simulink model "pendule_inverse"  (R2020b)
settings: Solver=ode5  StartTime=0.0  StopTime=20  FixedStep=0.1  RelTol=1e-3  EnableMultiTasking=on
values from neighbouring files (symbols this model uses):
  A = [ 0 1     0     0 ... (first row only)    [script_Labo4.m]
  B = [ 0 1/M 0 1/(M*l) ]'    [script_Labo4.m]
  g = 9.81    [script_Labo4.m]
  l = 0.5    [script_Labo4.m]
  m = 1    [script_Labo4.m]
  M = 1    [script_Labo4.m]
undefined symbols (not defined in the file or in its folder): Kd1, Kd2, Kp1, Kp2
settings Model: Creator=Administrateur  LastModifiedBy=dsaussie
settings SolverCC: AutoInsertRateTranBlk=on
settings DataIOCC: LimitDataPoints=on  SaveFormat=Array  SignalLoggingSaveFormat=ModelDataLogs  ReturnWorkspaceOutputs=off
settings OptimizationCC: ExpressionDepthLimit=2147483647  InitFltsAndDblsToZero=on  LifeSpan=inf
settings DebuggingCC: UnderspecifiedInitializationDetection=Classic  MergeDetectMultiDrivingBlocksExec=none  SolverPrmCheckMsg=warning  FcnCallInpInsideContextMsg=warning  StateNameClashWarn=warning  SFUnexpectedBacktrackingDiag=warning  SFNoUnconditionalDefaultTransitionDiag=warning  SFExecutionAtInitializationDiag=none  ArithmeticOperatorsInVariantConditions=warning
settings HardwareCC: ProdBitPerPointer=32  ProdBitPerSizeT=32  ProdBitPerPtrDiffT=32  ProdLargestAtomicFloat=None  ProdIntDivRoundTo=Undefined  ProdEndianess=Unspecified  ProdWordSize=32  ProdHWDeviceType=32-bit Generic
settings ModelReferenceCC: PropagateSignalLabelsOutOfModel=off
settings SFSimCC: SimUseLocalCustomCode=off  CustomCodeUndefinedFunction=UseInterfaceOnly
settings RTWCC: RTWUseLocalCustomCode=off
settings CodeAppCC: StateflowObjectComments=on
settings GRTTargetCC: TargetLangStandard=C89/C90 (ANSI)  CombineOutputUpdateFcns=off  GRTInterface=on
settings ConfigComp: CovMetricSettings=dw  CovSaveCumulativeToWorkspaceVar=on  CovSaveSingleToWorkspaceVar=on  CovExternalEMLEnable=off

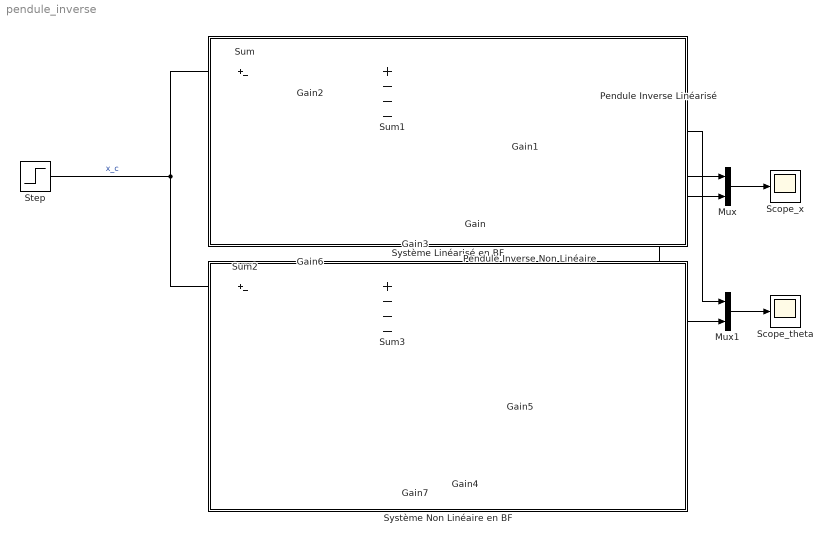
== system pendule_inverse ==
  Gain : Gain  Gain=Kp1
  Gain1 : Gain  Gain=Kd1
  Gain2 : Gain  Gain=Kp2
  Gain3 : Gain  Gain=Kd2
  Gain4 : Gain  Gain=Kp1
  Gain5 : Gain  Gain=Kd1
  Gain6 : Gain  Gain=Kp2
  Gain7 : Gain  Gain=Kd2
  Mux : Mux  Inputs=2
  Mux1 : Mux  Inputs=2
  Pendule Inverse Linéarisé : Subsystem
  Pendule Inverse Non Linéaire : Subsystem
  Scope_theta : Scope
  Scope_x : Scope
  Step : Step  Time=0  SampleTime=0
  Sum : Sum  Inputs=|+-
  Sum1 : Sum  Inputs=+---
  Sum2 : Sum  Inputs=|+-
  Sum3 : Sum  Inputs=+---
  Système Linéarisé en BF : Subsystem
  Système Non Linéaire en BF : Subsystem
  wires:
  Pendule Inverse Non Linéaire/1(x) -> Mux/2, Sum2/2
  Pendule Inverse Non Linéaire/3("theta ") -> Mux1/2, Gain4/1
  Sum3/1 -> Pendule Inverse Non Linéaire/1(u)
  Pendule Inverse Non Linéaire/2("x_dot ") -> Gain7/1
  Pendule Inverse Non Linéaire/4("theta_dot ") -> Gain5/1
  Step/1 -> Sum/1, Sum2/1  "x_c"
  Sum1/1 -> Pendule Inverse Linéarisé/1(delta_u)
  Pendule Inverse Linéarisé/4(delta_theta_dot) -> Gain1/1
  Pendule Inverse Linéarisé/3(delta_theta) -> Gain/1, Mux1/1
  Sum/1 -> Gain2/1
  Gain2/1 -> Sum1/1
  Pendule Inverse Linéarisé/2(delta_x_dot) -> Gain3/1
  Gain1/1 -> Sum1/4
  Gain/1 -> Sum1/3
  Gain3/1 -> Sum1/2
  Pendule Inverse Linéarisé/1(delta_x) -> Mux/1, Sum/2
  Gain7/1 -> Sum3/2
  Gain4/1 -> Sum3/3
  Gain5/1 -> Sum3/4
  Gain6/1 -> Sum3/1
  Sum2/1 -> Gain6/1
  Mux/1 -> Scope_x/1
  Mux1/1 -> Scope_theta/1

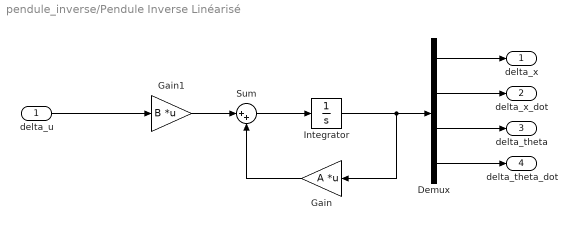
== system pendule_inverse/Pendule Inverse Linéarisé ==
  delta_u : Inport
  Demux : Demux
  Gain : Gain  Gain=A  Multiplication=Matrix(K*u)
  Gain1 : Gain  Gain=B  Multiplication=Matrix(K*u)
  Integrator : Integrator
  Sum : Sum  Inputs=|++
  delta_x : Outport
  delta_x_dot : Outport  Port=2
  delta_theta : Outport  Port=3
  delta_theta_dot : Outport  Port=4
  wires:
  Demux/4 -> delta_theta_dot/1
  delta_u/1 -> Gain1/1
  Sum/1 -> Integrator/1
  Integrator/1 -> Demux/1, Gain/1
  Demux/3 -> delta_theta/1
  Demux/1 -> delta_x/1
  Demux/2 -> delta_x_dot/1
  Gain/1 -> Sum/2
  Gain1/1 -> Sum/1

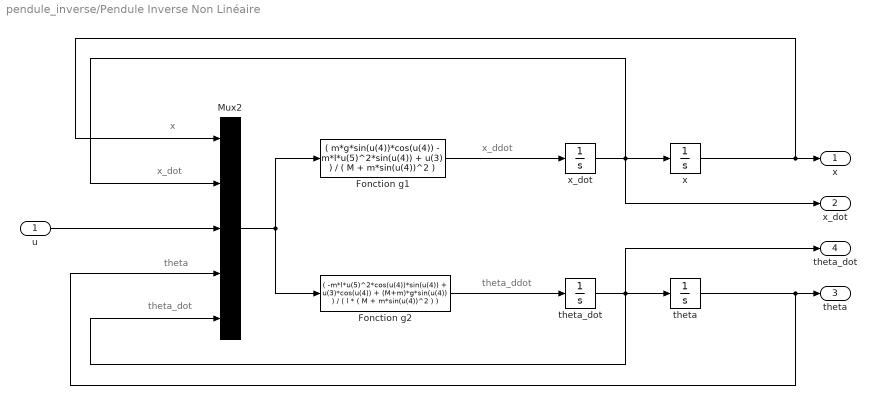
== system pendule_inverse/Pendule Inverse Non Linéaire ==
  note: x
  note: x_dot
  note: theta
  note: theta_dot
  note: x_ddot
  note: theta_ddot
  u : Inport
  " theta_dot" : Integrator
  " x_dot" : Integrator
  Fonction g1 : Fcn  Expr="( m*g*sin(u(4))*cos(u(4)) - m*l*u(5)^2*sin(u(4)) + u(3) ) / ( M + m*sin(u(4))^2  )"
  Fonction g2 : Fcn  Expr="( -m*l*u(5)^2*cos(u(4))*sin(u(4)) + u(3)*cos(u(4)) + (M+m)*g*sin(u(4)) ) / (  l * ( M + m*sin(u(4))^2 )  )"
  Mux2 : Mux  Inputs=5
  theta : Integrator  LimitOutput=on  UpperSaturationLimit=pi/2  LowerSaturationLimit=-pi/2
  "x " : Integrator  LowerSaturationLimit=-9.5
  x : Outport
  "x_dot " : Outport  Port=2
  "theta " : Outport  Port=3
  "theta_dot " : Outport  Port=4
  wires:
  Fonction g1/1 -> " x_dot"/1
  " x_dot"/1 -> "x_dot "/1, Mux2/2, "x "/1
  Mux2/1 -> Fonction g1/1, Fonction g2/1
  Fonction g2/1 -> " theta_dot"/1
  u/1 -> Mux2/3
  " theta_dot"/1 -> "theta_dot "/1, Mux2/5, theta/1
  theta/1 -> "theta "/1, Mux2/4
  "x "/1 -> x/1, Mux2/1

== system pendule_inverse/Système Linéarisé en BF ==

== system pendule_inverse/Système Non Linéaire en BF ==
